simulink model "SPMeT_CCCV_chrg_controller"  (R2019a)
settings: Solver=VariableStepAuto  StartTime=0.0  StopTime=10.0  RelTol=1e-3
libraries: simulink x1
settings Model: Creator=ztakeo  LastModifiedBy=ztakeo

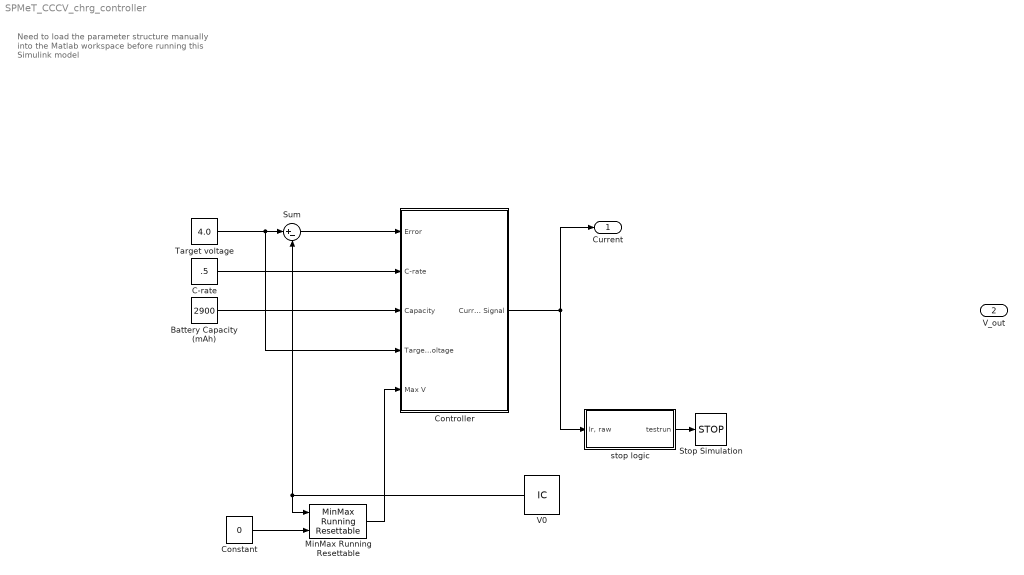
== system SPMeT_CCCV_chrg_controller ==
  note: Need to load the parameter structure manually into the Matlab workspace before running this Simulink model
  Battery Capacity (mAh) : Constant  Value=2900  OutDataTypeStr=double
  C-rate : Constant  Value=.5  OutDataTypeStr=double
  Constant : Constant  Value=0
  Controller : Subsystem
  MinMax Running Resettable : simulink/Math Operations/MinMax Running Resettable  Function=max  vinit=0.0
  Stop Simulation : Stop
  Sum : Sum  Inputs=|+-
  "Target voltage " : Constant  Value=4.0  OutDataTypeStr=double
  V0 : InitialCondition  Value=2.8
  stop logic : Subsystem
  Current : Outport
  "V_out " : Outport  Port=2
  wires:
  Sum/1 -> Controller/1(Error)
  Controller/1(Current Signal) -> Current/1, stop logic/1("Ir, raw ")
  Constant/1 -> MinMax Running Resettable/2
  "Target voltage "/1 -> Controller/4(Target Voltage), Sum/1
  MinMax Running Resettable/1 -> Controller/5(Max V)
  C-rate/1 -> Controller/2(C-rate)
  Battery Capacity (mAh)/1 -> Controller/3(Capacity)
  ? -> V0/1, "V_out "/1
  stop logic/1(testrun) -> Stop Simulation/1
  V0/1 -> Sum/2, MinMax Running Resettable/1

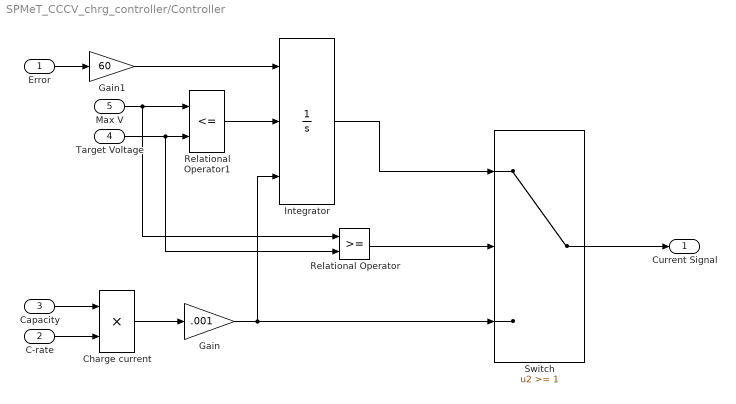
== system SPMeT_CCCV_chrg_controller/Controller ==
  Error : Inport
  C-rate : Inport  Port=2
  Capacity : Inport  Port=3
  Target Voltage : Inport  Port=4
  Max V : Inport  Port=5
  Charge current : Product
  Gain : Gain  Gain=.001
  Gain1 : Gain  Gain=60
  Integrator : Integrator  ExternalReset=level  InitialConditionSource=external
  Relational Operator : RelationalOperator  OutDataTypeStr=boolean  RndMeth=Nearest
  Relational Operator1 : RelationalOperator  Operator=<=  OutDataTypeStr=boolean  RndMeth=Nearest
  Switch : Switch  Threshold=1
  Current Signal : Outport
  wires:
  Error/1 -> Gain1/1
  Target Voltage/1 -> Relational Operator/2, Relational Operator1/2
  Switch/1 -> Current Signal/1
  C-rate/1 -> Charge current/2
  Capacity/1 -> Charge current/1
  Gain/1 -> Switch/3, Integrator/3
  Relational Operator1/1 -> Integrator/2
  Max V/1 -> Relational Operator/1, Relational Operator1/1
  Gain1/1 -> Integrator/1
  Charge current/1 -> Gain/1
  Integrator/1 -> Switch/1
  Relational Operator/1 -> Switch/2

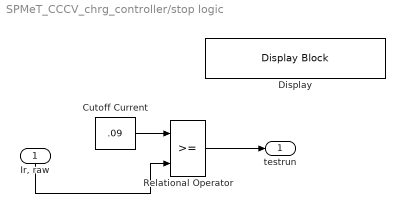
== system SPMeT_CCCV_chrg_controller/stop logic ==
  "Ir, raw " : Inport
  Cutoff Current : Constant  Value=.09  OutDataTypeStr=double
  Display : DisplayBlock  LabelPosition=Hide  Format=short
  Relational Operator : RelationalOperator  OutDataTypeStr=boolean  RndMeth=Nearest
  testrun : Outport
  wires:
  Cutoff Current/1 -> Relational Operator/1
  Relational Operator/1 -> testrun/1
  "Ir, raw "/1 -> Relational Operator/2
